simulink model "UDPSend"  (R2016b)
settings: Solver=FixedStepDiscrete  StartTime=0.0  StopTime=10.0  FixedStep=1e-3  RelTol=1e-3
libraries: mbed_ethernet_udp x3, simulink x1, mbed_lib x1
settings Model: Creator=oh  LastModifiedBy=oh
settings OptimizationCC: DefaultParameterBehavior=Inlined
settings DebuggingCC: ParameterTunabilityLossMsg=error
settings HardwareCC: ProdBitPerPointer=32  ProdBitPerSizeT=32  ProdBitPerPtrDiffT=32  ProdLargestAtomicInteger=Long  ProdLargestAtomicFloat=Double  ProdWordSize=32  ProdHWDeviceType=ARM Compatible->ARM Cortex
settings RTWCC: SystemTargetFile=mbed.tlc  TemplateMakefile=mbed.tmf  Description=MbedTarget (Embedded Target for Embedded Coder)  IncludeHyperlinkInReport=on  TargetLang=C++
settings CodeAppCC: ForceParamTrailComments=on  IgnoreCustomStorageClasses=off  OperatorAnnotations=on  SimulinkDataObjDesc=on  SFDataObjDesc=on  MATLABFcnDesc=on  InsertBlockDesc=on  MATLABSourceComments=on
settings STFCustomTargetCC: TargetLibSuffix=.a  TargetLangStandard=C++03 (ISO)  GenerateSampleERTMain=on  CombineOutputUpdateFcns=on  ERTCustomFileBanners=on  SupportContinuousTime=off  SupportNonInlinedSFcns=off  RemoveResetFunc=on  MATLABClassNameForMDSCustomization=Simulink.SoftwareTarget.ERTCustomization  ModelStepFunctionPrototypeControlCompliant=on  GRTInterface=off  SystemTargetFile=mbed.tlc
settings ERTTargetCC: TargetLangStandard=C++03 (ISO)  GenerateSampleERTMain=on  ParMdlRefBuildCompliant=off  CompOptLevelCompliant=off  ConcurrentExecutionCompliant=off  ERTFirstTimeCompliant=off  CPPClassGenCompliant=off  UseToolchainInfoCompliant=off  InlinedParameterPlacement=NonHierarchical  ERTCustomFileTemplate=mbed_file_process.tlc

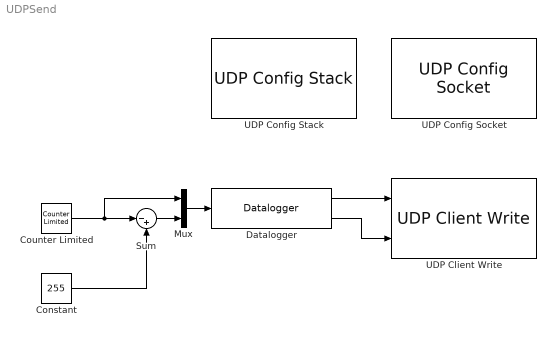
== system UDPSend ==
  Constant : Constant  Value=255  OutDataTypeStr=uint8
  Counter Limited : simulink/Sources/Counter Limited  uplimit=255  tsamp=1
  Datalogger : mbed_lib/Utilities/Datalogger  TypeInputPorts={ 'uint8' 2 }  TypeOfInputs={'2*uint8'}  BufferSize=100  errEn=off  SampleTime=-1
  Mux : Mux  Inputs=2
  Sum : Sum  Inputs=|-+
  UDP Client Write : mbed_ethernet_udp/UDP Client Write  sock_ID=1  numData=on  SampleTime=-1
  UDP Config Socket : mbed_ethernet_udp/UDP Config Socket  Priority=1  des_IP='192.168.178.20'  des_port=10001  sock_ID=1
  UDP Config Stack : mbed_ethernet_udp/UDP Config Stack  Priority=0  sDHCP=off  DHCP=0  ip_addr='192.168.178.200'  sub_mask='255.255.255.0'  gateway='0.0.0.0'
  wires:
  Datalogger/1 -> UDP Client Write/1
  Datalogger/2 -> UDP Client Write/2
  Counter Limited/1 -> Mux/1, Sum/1
  Constant/1 -> Sum/2
  Mux/1 -> Datalogger/1
  Sum/1 -> Mux/2
